simulink model "TST_AccPed_DrvDemStpLim"  (R2016b)
settings: Solver=FixedStepDiscrete  StartTime=0.0  StopTime=simTime  FixedStep=sampleTime  RelTol=1e-3
values from neighbouring files (symbols this model uses):
  testCase = 1    [initTST_AccPed_DrvDemStpLim_001.m]    (also in initTST_AccPed_DrvDemStpLim_002.m = 2; initTST_AccPed_DrvDemStpLim_003.m = 3)
libraries: simulink x13, UnitTest_Lib x9
settings Model: Creator=zhengjinyan  LastModifiedBy=zhengjinyan
settings DebuggingCC: SignalRangeChecking=error

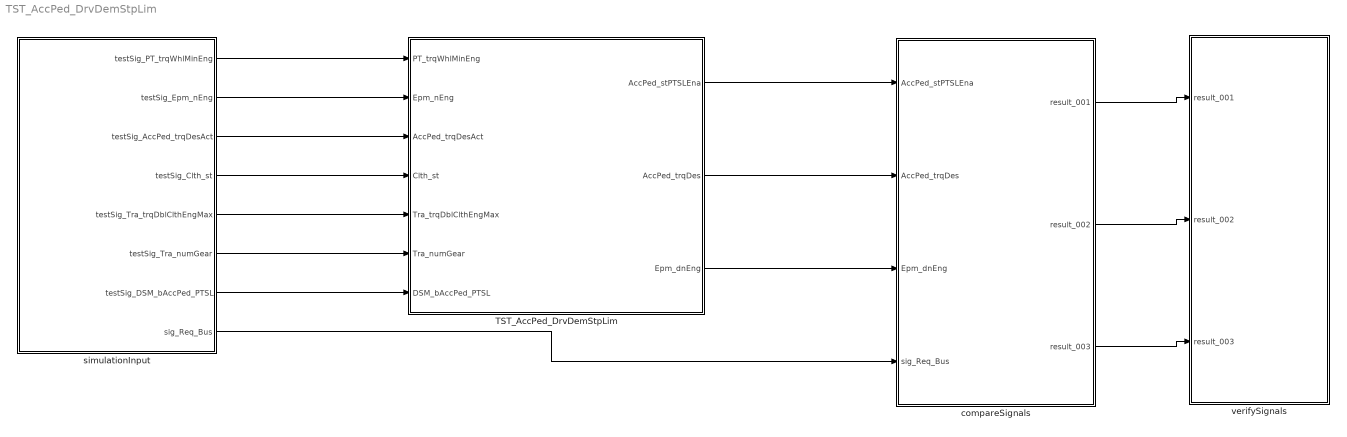
== system TST_AccPed_DrvDemStpLim ==
  TST_AccPed_DrvDemStpLim : Subsystem
  compareSignals : Subsystem
  simulationInput : Subsystem
  verifySignals : Subsystem
  wires:
  simulationInput/1(testSig_PT_trqWhlMinEng) -> TST_AccPed_DrvDemStpLim/1(PT_trqWhlMinEng)
  simulationInput/2(testSig_Epm_nEng) -> TST_AccPed_DrvDemStpLim/2(Epm_nEng)
  simulationInput/3(testSig_AccPed_trqDesAct) -> TST_AccPed_DrvDemStpLim/3(AccPed_trqDesAct)
  simulationInput/4(testSig_Clth_st) -> TST_AccPed_DrvDemStpLim/4(Clth_st)
  simulationInput/5(testSig_Tra_trqDblClthEngMax) -> TST_AccPed_DrvDemStpLim/5(Tra_trqDblClthEngMax)
  simulationInput/6(testSig_Tra_numGear) -> TST_AccPed_DrvDemStpLim/6(Tra_numGear)
  simulationInput/7(testSig_DSM_bAccPed_PTSL) -> TST_AccPed_DrvDemStpLim/7(DSM_bAccPed_PTSL)
  TST_AccPed_DrvDemStpLim/1(AccPed_stPTSLEna) -> compareSignals/1(AccPed_stPTSLEna)
  TST_AccPed_DrvDemStpLim/2(AccPed_trqDes) -> compareSignals/2(AccPed_trqDes)
  TST_AccPed_DrvDemStpLim/3(Epm_dnEng) -> compareSignals/3(Epm_dnEng)
  simulationInput/8(sig_Req_Bus) -> compareSignals/4(sig_Req_Bus)
  compareSignals/1(result_001) -> verifySignals/1(result_001)
  compareSignals/2(result_002) -> verifySignals/2(result_002)
  compareSignals/3(result_003) -> verifySignals/3(result_003)

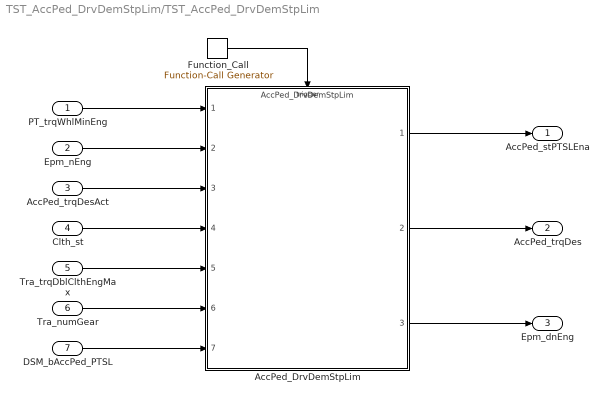
== system TST_AccPed_DrvDemStpLim/TST_AccPed_DrvDemStpLim ==
  PT_trqWhlMinEng : Inport
  Epm_nEng : Inport  Port=2
  AccPed_trqDesAct : Inport  Port=3
  Clth_st : Inport  Port=4
  Tra_trqDblClthEngMax : Inport  Port=5
  Tra_numGear : Inport  Port=6
  DSM_bAccPed_PTSL : Inport  Port=7
  AccPed_DrvDemStpLim : ModelReference  ModelNameDialog=AccPed_DrvDemStpLim  SimulationMode=Normal  ModelReferenceVersion=1.9  TriggerPortName=function  TriggerPortTriggerType=function-call  TriggerPortStatesWhenEnabling=held
  Function_Call : simulink/Ports & Subsystems/Function-Call Generator  sample_time=sampleTime  numberOfIterations=1
  AccPed_stPTSLEna : Outport
  AccPed_trqDes : Outport  Port=2
  Epm_dnEng : Outport  Port=3
  wires:
  Function_Call/1 -> AccPed_DrvDemStpLim/Trigger
  PT_trqWhlMinEng/1 -> AccPed_DrvDemStpLim/1
  Epm_nEng/1 -> AccPed_DrvDemStpLim/2
  AccPed_trqDesAct/1 -> AccPed_DrvDemStpLim/3
  Clth_st/1 -> AccPed_DrvDemStpLim/4
  Tra_trqDblClthEngMax/1 -> AccPed_DrvDemStpLim/5
  Tra_numGear/1 -> AccPed_DrvDemStpLim/6
  DSM_bAccPed_PTSL/1 -> AccPed_DrvDemStpLim/7
  AccPed_DrvDemStpLim/1 -> AccPed_stPTSLEna/1
  AccPed_DrvDemStpLim/2 -> AccPed_trqDes/1
  AccPed_DrvDemStpLim/3 -> Epm_dnEng/1

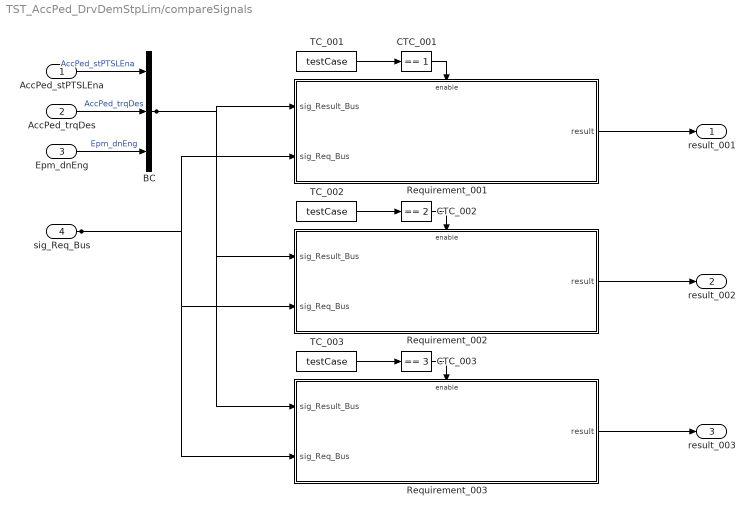
== system TST_AccPed_DrvDemStpLim/compareSignals ==
  AccPed_stPTSLEna : Inport
  AccPed_trqDes : Inport  Port=2
  Epm_dnEng : Inport  Port=3
  sig_Req_Bus : Inport  Port=4
  BC : BusCreator  Inputs=3
  CTC_001 : simulink/Logic and Bit Operations/Compare To Constant  relop===  const=1  OutDataTypeStr=boolean
  CTC_002 : simulink/Logic and Bit Operations/Compare To Constant  relop===  const=2  OutDataTypeStr=boolean
  CTC_003 : simulink/Logic and Bit Operations/Compare To Constant  relop===  const=3  OutDataTypeStr=boolean
  Requirement_001 : Subsystem
  Requirement_002 : Subsystem
  Requirement_003 : Subsystem
  TC_001 : Constant  Value=testCase
  TC_002 : Constant  Value=testCase
  TC_003 : Constant  Value=testCase
  result_001 : Outport
  result_002 : Outport  Port=2
  result_003 : Outport  Port=3
  wires:
  AccPed_stPTSLEna/1 -> BC/1  "AccPed_stPTSLEna"
  AccPed_trqDes/1 -> BC/2  "AccPed_trqDes"
  Epm_dnEng/1 -> BC/3  "Epm_dnEng"
  TC_001/1 -> CTC_001/1
  CTC_001/1 -> Requirement_001/Enable
  sig_Req_Bus/1 -> Requirement_001/2(sig_Req_Bus), Requirement_002/2(sig_Req_Bus), Requirement_003/2(sig_Req_Bus)
  BC/1 -> Requirement_001/1(sig_Result_Bus), Requirement_002/1(sig_Result_Bus), Requirement_003/1(sig_Result_Bus)
  Requirement_001/1(result) -> result_001/1
  TC_002/1 -> CTC_002/1
  CTC_002/1 -> Requirement_002/Enable
  Requirement_002/1(result) -> result_002/1
  TC_003/1 -> CTC_003/1
  CTC_003/1 -> Requirement_003/Enable
  Requirement_003/1(result) -> result_003/1

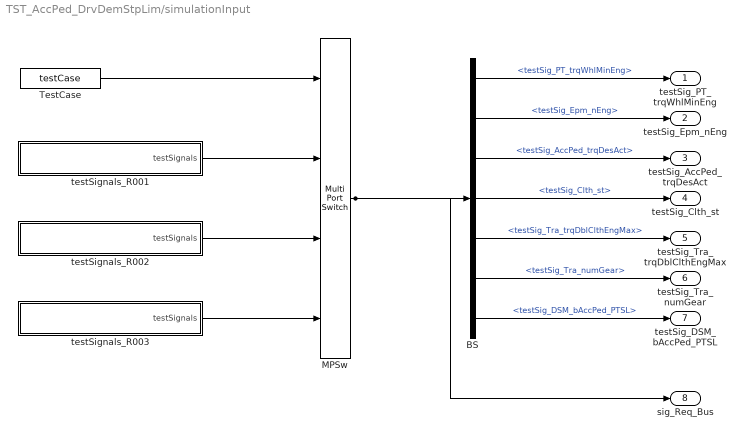
== system TST_AccPed_DrvDemStpLim/simulationInput ==
  BS : BusSelector  OutputSignals=testSig_PT_trqWhlMinEng,testSig_Epm_nEng,testSig_AccPed_trqDesAct,testSig_Clth_st,testSig_Tra_trqDblClthEngMax,testSig_Tra_numGear,testSig_DSM_bAccPed_PTSL
  MPSw : MultiPortSwitch  SaturateOnIntegerOverflow=on  InputSameDT=on
  TestCase : Constant  Value=testCase
  testSignals_R001 : Subsystem
  testSignals_R002 : Subsystem
  testSignals_R003 : Subsystem
  testSig_PT_trqWhlMinEng : Outport
  testSig_Epm_nEng : Outport  Port=2
  testSig_AccPed_trqDesAct : Outport  Port=3
  testSig_Clth_st : Outport  Port=4
  testSig_Tra_trqDblClthEngMax : Outport  Port=5
  testSig_Tra_numGear : Outport  Port=6
  testSig_DSM_bAccPed_PTSL : Outport  Port=7
  sig_Req_Bus : Outport  Port=8
  wires:
  BS/1 -> testSig_PT_trqWhlMinEng/1  "<testSig_PT_trqWhlMinEng>"
  BS/2 -> testSig_Epm_nEng/1  "<testSig_Epm_nEng>"
  BS/3 -> testSig_AccPed_trqDesAct/1  "<testSig_AccPed_trqDesAct>"
  BS/4 -> testSig_Clth_st/1  "<testSig_Clth_st>"
  BS/5 -> testSig_Tra_trqDblClthEngMax/1  "<testSig_Tra_trqDblClthEngMax>"
  BS/6 -> testSig_Tra_numGear/1  "<testSig_Tra_numGear>"
  BS/7 -> testSig_DSM_bAccPed_PTSL/1  "<testSig_DSM_bAccPed_PTSL>"
  MPSw/1 -> BS/1, sig_Req_Bus/1
  TestCase/1 -> MPSw/1
  testSignals_R001/1(testSignals) -> MPSw/2
  testSignals_R002/1(testSignals) -> MPSw/3
  testSignals_R003/1(testSignals) -> MPSw/4

== system TST_AccPed_DrvDemStpLim/verifySignals ==
  result_001 : Inport
  result_002 : Inport  Port=2
  result_003 : Inport  Port=3
  Assertion_001 : Assertion  Enabled=off
  Assertion_002 : Assertion  Enabled=off
  Assertion_003 : Assertion  Enabled=off
  wires:
  result_001/1 -> Assertion_001/1
  result_002/1 -> Assertion_002/1
  result_003/1 -> Assertion_003/1

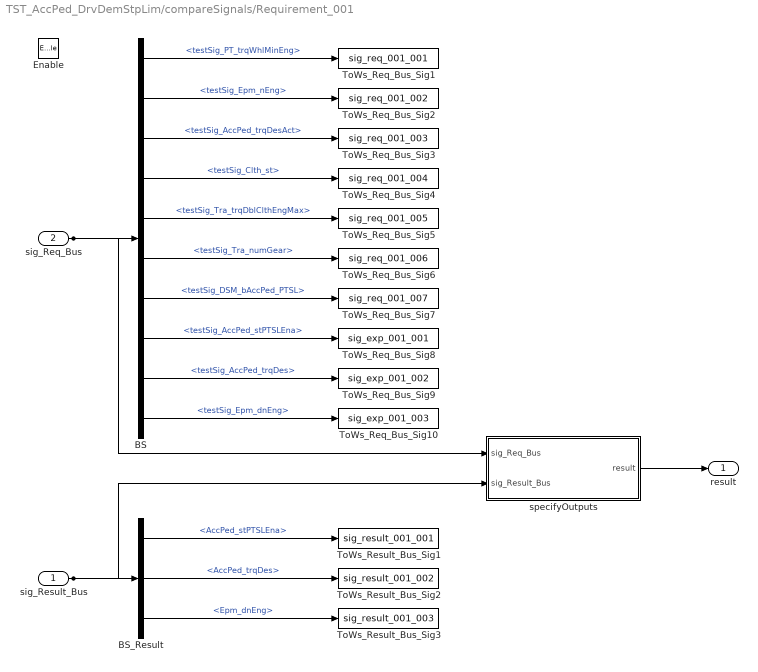
== system TST_AccPed_DrvDemStpLim/compareSignals/Requirement_001 ==
  sig_Result_Bus : Inport
  sig_Req_Bus : Inport  Port=2
  Enable : EnablePort
  BS : BusSelector  OutputSignals=testSig_PT_trqWhlMinEng,testSig_Epm_nEng,testSig_AccPed_trqDesAct,testSig_Clth_st,testSig_Tra_trqDblClthEngMax,testSig_Tra_numGear,testSig_DSM_bAccPed_PTSL,testSig_AccPed_stPTSLEna,testSig_AccPed_trqDes,testSig_Epm_dnEng
  BS_Result : BusSelector  OutputSignals=AccPed_stPTSLEna,AccPed_trqDes,Epm_dnEng
  ToWs_Req_Bus_Sig1 : ToWorkspace  VariableName=sig_req_001_001  SaveFormat=Structure With Time
  ToWs_Req_Bus_Sig10 : ToWorkspace  VariableName=sig_exp_001_003  SaveFormat=Structure With Time
  ToWs_Req_Bus_Sig2 : ToWorkspace  VariableName=sig_req_001_002  SaveFormat=Structure With Time
  ToWs_Req_Bus_Sig3 : ToWorkspace  VariableName=sig_req_001_003  SaveFormat=Structure With Time
  ToWs_Req_Bus_Sig4 : ToWorkspace  VariableName=sig_req_001_004  SaveFormat=Structure With Time
  ToWs_Req_Bus_Sig5 : ToWorkspace  VariableName=sig_req_001_005  SaveFormat=Structure With Time
  ToWs_Req_Bus_Sig6 : ToWorkspace  VariableName=sig_req_001_006  SaveFormat=Structure With Time
  ToWs_Req_Bus_Sig7 : ToWorkspace  VariableName=sig_req_001_007  SaveFormat=Structure With Time
  ToWs_Req_Bus_Sig8 : ToWorkspace  VariableName=sig_exp_001_001  SaveFormat=Structure With Time
  ToWs_Req_Bus_Sig9 : ToWorkspace  VariableName=sig_exp_001_002  SaveFormat=Structure With Time
  ToWs_Result_Bus_Sig1 : ToWorkspace  VariableName=sig_result_001_001  SaveFormat=Structure With Time
  ToWs_Result_Bus_Sig2 : ToWorkspace  VariableName=sig_result_001_002  SaveFormat=Structure With Time
  ToWs_Result_Bus_Sig3 : ToWorkspace  VariableName=sig_result_001_003  SaveFormat=Structure With Time
  specifyOutputs : Subsystem
  result : Outport
  wires:
  sig_Req_Bus/1 -> BS/1, specifyOutputs/1(sig_Req_Bus)
  BS/1 -> ToWs_Req_Bus_Sig1/1  "<testSig_PT_trqWhlMinEng>"
  BS/2 -> ToWs_Req_Bus_Sig2/1  "<testSig_Epm_nEng>"
  BS/3 -> ToWs_Req_Bus_Sig3/1  "<testSig_AccPed_trqDesAct>"
  BS/4 -> ToWs_Req_Bus_Sig4/1  "<testSig_Clth_st>"
  BS/5 -> ToWs_Req_Bus_Sig5/1  "<testSig_Tra_trqDblClthEngMax>"
  BS/6 -> ToWs_Req_Bus_Sig6/1  "<testSig_Tra_numGear>"
  BS/7 -> ToWs_Req_Bus_Sig7/1  "<testSig_DSM_bAccPed_PTSL>"
  BS/8 -> ToWs_Req_Bus_Sig8/1  "<testSig_AccPed_stPTSLEna>"
  BS/9 -> ToWs_Req_Bus_Sig9/1  "<testSig_AccPed_trqDes>"
  BS/10 -> ToWs_Req_Bus_Sig10/1  "<testSig_Epm_dnEng>"
  sig_Result_Bus/1 -> BS_Result/1, specifyOutputs/2(sig_Result_Bus)
  BS_Result/1 -> ToWs_Result_Bus_Sig1/1  "<AccPed_stPTSLEna>"
  BS_Result/2 -> ToWs_Result_Bus_Sig2/1  "<AccPed_trqDes>"
  BS_Result/3 -> ToWs_Result_Bus_Sig3/1  "<Epm_dnEng>"
  specifyOutputs/1(result) -> result/1

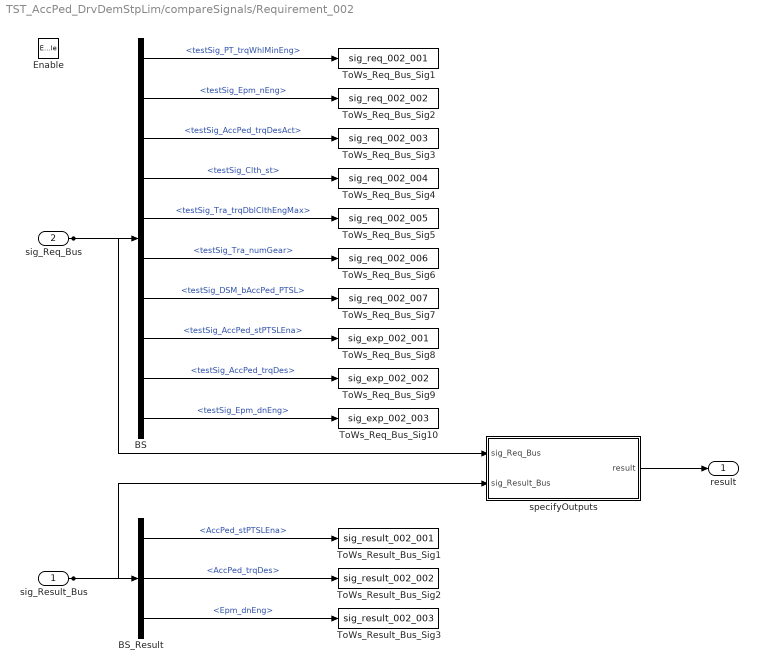
== system TST_AccPed_DrvDemStpLim/compareSignals/Requirement_002 ==
  sig_Result_Bus : Inport
  sig_Req_Bus : Inport  Port=2
  Enable : EnablePort
  BS : BusSelector  OutputSignals=testSig_PT_trqWhlMinEng,testSig_Epm_nEng,testSig_AccPed_trqDesAct,testSig_Clth_st,testSig_Tra_trqDblClthEngMax,testSig_Tra_numGear,testSig_DSM_bAccPed_PTSL,testSig_AccPed_stPTSLEna,testSig_AccPed_trqDes,testSig_Epm_dnEng
  BS_Result : BusSelector  OutputSignals=AccPed_stPTSLEna,AccPed_trqDes,Epm_dnEng
  ToWs_Req_Bus_Sig1 : ToWorkspace  VariableName=sig_req_002_001  SaveFormat=Structure With Time
  ToWs_Req_Bus_Sig10 : ToWorkspace  VariableName=sig_exp_002_003  SaveFormat=Structure With Time
  ToWs_Req_Bus_Sig2 : ToWorkspace  VariableName=sig_req_002_002  SaveFormat=Structure With Time
  ToWs_Req_Bus_Sig3 : ToWorkspace  VariableName=sig_req_002_003  SaveFormat=Structure With Time
  ToWs_Req_Bus_Sig4 : ToWorkspace  VariableName=sig_req_002_004  SaveFormat=Structure With Time
  ToWs_Req_Bus_Sig5 : ToWorkspace  VariableName=sig_req_002_005  SaveFormat=Structure With Time
  ToWs_Req_Bus_Sig6 : ToWorkspace  VariableName=sig_req_002_006  SaveFormat=Structure With Time
  ToWs_Req_Bus_Sig7 : ToWorkspace  VariableName=sig_req_002_007  SaveFormat=Structure With Time
  ToWs_Req_Bus_Sig8 : ToWorkspace  VariableName=sig_exp_002_001  SaveFormat=Structure With Time
  ToWs_Req_Bus_Sig9 : ToWorkspace  VariableName=sig_exp_002_002  SaveFormat=Structure With Time
  ToWs_Result_Bus_Sig1 : ToWorkspace  VariableName=sig_result_002_001  SaveFormat=Structure With Time
  ToWs_Result_Bus_Sig2 : ToWorkspace  VariableName=sig_result_002_002  SaveFormat=Structure With Time
  ToWs_Result_Bus_Sig3 : ToWorkspace  VariableName=sig_result_002_003  SaveFormat=Structure With Time
  specifyOutputs : Subsystem
  result : Outport
  wires:
  sig_Req_Bus/1 -> BS/1, specifyOutputs/1(sig_Req_Bus)
  BS/1 -> ToWs_Req_Bus_Sig1/1  "<testSig_PT_trqWhlMinEng>"
  BS/2 -> ToWs_Req_Bus_Sig2/1  "<testSig_Epm_nEng>"
  BS/3 -> ToWs_Req_Bus_Sig3/1  "<testSig_AccPed_trqDesAct>"
  BS/4 -> ToWs_Req_Bus_Sig4/1  "<testSig_Clth_st>"
  BS/5 -> ToWs_Req_Bus_Sig5/1  "<testSig_Tra_trqDblClthEngMax>"
  BS/6 -> ToWs_Req_Bus_Sig6/1  "<testSig_Tra_numGear>"
  BS/7 -> ToWs_Req_Bus_Sig7/1  "<testSig_DSM_bAccPed_PTSL>"
  BS/8 -> ToWs_Req_Bus_Sig8/1  "<testSig_AccPed_stPTSLEna>"
  BS/9 -> ToWs_Req_Bus_Sig9/1  "<testSig_AccPed_trqDes>"
  BS/10 -> ToWs_Req_Bus_Sig10/1  "<testSig_Epm_dnEng>"
  sig_Result_Bus/1 -> BS_Result/1, specifyOutputs/2(sig_Result_Bus)
  BS_Result/1 -> ToWs_Result_Bus_Sig1/1  "<AccPed_stPTSLEna>"
  BS_Result/2 -> ToWs_Result_Bus_Sig2/1  "<AccPed_trqDes>"
  BS_Result/3 -> ToWs_Result_Bus_Sig3/1  "<Epm_dnEng>"
  specifyOutputs/1(result) -> result/1

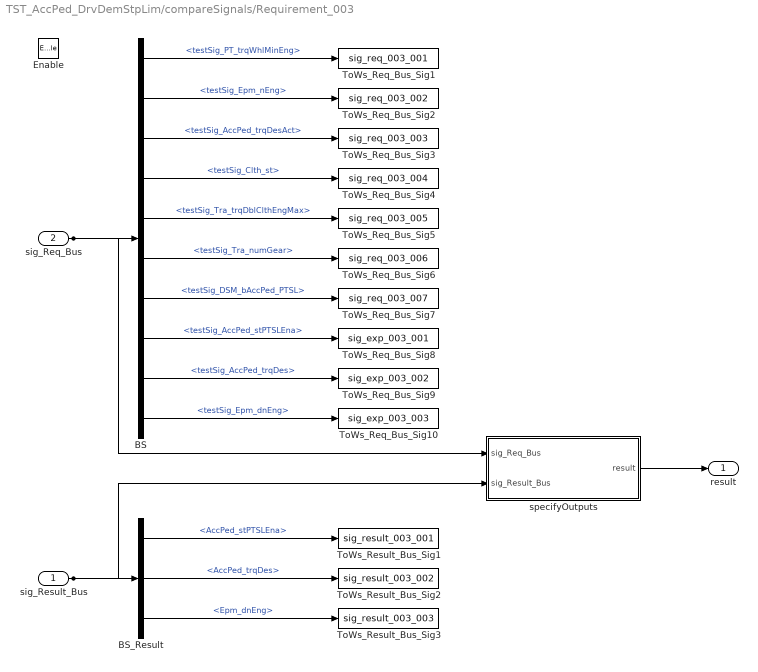
== system TST_AccPed_DrvDemStpLim/compareSignals/Requirement_003 ==
  sig_Result_Bus : Inport
  sig_Req_Bus : Inport  Port=2
  Enable : EnablePort
  BS : BusSelector  OutputSignals=testSig_PT_trqWhlMinEng,testSig_Epm_nEng,testSig_AccPed_trqDesAct,testSig_Clth_st,testSig_Tra_trqDblClthEngMax,testSig_Tra_numGear,testSig_DSM_bAccPed_PTSL,testSig_AccPed_stPTSLEna,testSig_AccPed_trqDes,testSig_Epm_dnEng
  BS_Result : BusSelector  OutputSignals=AccPed_stPTSLEna,AccPed_trqDes,Epm_dnEng
  ToWs_Req_Bus_Sig1 : ToWorkspace  VariableName=sig_req_003_001  SaveFormat=Structure With Time
  ToWs_Req_Bus_Sig10 : ToWorkspace  VariableName=sig_exp_003_003  SaveFormat=Structure With Time
  ToWs_Req_Bus_Sig2 : ToWorkspace  VariableName=sig_req_003_002  SaveFormat=Structure With Time
  ToWs_Req_Bus_Sig3 : ToWorkspace  VariableName=sig_req_003_003  SaveFormat=Structure With Time
  ToWs_Req_Bus_Sig4 : ToWorkspace  VariableName=sig_req_003_004  SaveFormat=Structure With Time
  ToWs_Req_Bus_Sig5 : ToWorkspace  VariableName=sig_req_003_005  SaveFormat=Structure With Time
  ToWs_Req_Bus_Sig6 : ToWorkspace  VariableName=sig_req_003_006  SaveFormat=Structure With Time
  ToWs_Req_Bus_Sig7 : ToWorkspace  VariableName=sig_req_003_007  SaveFormat=Structure With Time
  ToWs_Req_Bus_Sig8 : ToWorkspace  VariableName=sig_exp_003_001  SaveFormat=Structure With Time
  ToWs_Req_Bus_Sig9 : ToWorkspace  VariableName=sig_exp_003_002  SaveFormat=Structure With Time
  ToWs_Result_Bus_Sig1 : ToWorkspace  VariableName=sig_result_003_001  SaveFormat=Structure With Time
  ToWs_Result_Bus_Sig2 : ToWorkspace  VariableName=sig_result_003_002  SaveFormat=Structure With Time
  ToWs_Result_Bus_Sig3 : ToWorkspace  VariableName=sig_result_003_003  SaveFormat=Structure With Time
  specifyOutputs : Subsystem
  result : Outport
  wires:
  sig_Req_Bus/1 -> BS/1, specifyOutputs/1(sig_Req_Bus)
  BS/1 -> ToWs_Req_Bus_Sig1/1  "<testSig_PT_trqWhlMinEng>"
  BS/2 -> ToWs_Req_Bus_Sig2/1  "<testSig_Epm_nEng>"
  BS/3 -> ToWs_Req_Bus_Sig3/1  "<testSig_AccPed_trqDesAct>"
  BS/4 -> ToWs_Req_Bus_Sig4/1  "<testSig_Clth_st>"
  BS/5 -> ToWs_Req_Bus_Sig5/1  "<testSig_Tra_trqDblClthEngMax>"
  BS/6 -> ToWs_Req_Bus_Sig6/1  "<testSig_Tra_numGear>"
  BS/7 -> ToWs_Req_Bus_Sig7/1  "<testSig_DSM_bAccPed_PTSL>"
  BS/8 -> ToWs_Req_Bus_Sig8/1  "<testSig_AccPed_stPTSLEna>"
  BS/9 -> ToWs_Req_Bus_Sig9/1  "<testSig_AccPed_trqDes>"
  BS/10 -> ToWs_Req_Bus_Sig10/1  "<testSig_Epm_dnEng>"
  sig_Result_Bus/1 -> BS_Result/1, specifyOutputs/2(sig_Result_Bus)
  BS_Result/1 -> ToWs_Result_Bus_Sig1/1  "<AccPed_stPTSLEna>"
  BS_Result/2 -> ToWs_Result_Bus_Sig2/1  "<AccPed_trqDes>"
  BS_Result/3 -> ToWs_Result_Bus_Sig3/1  "<Epm_dnEng>"
  specifyOutputs/1(result) -> result/1

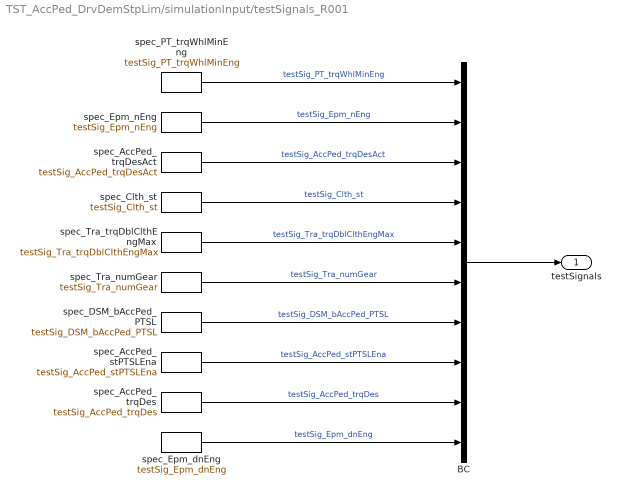
== system TST_AccPed_DrvDemStpLim/simulationInput/testSignals_R001 ==
  BC : BusCreator  Inputs=10
  spec_AccPed_stPTSLEna : FromWorkspace  VariableName=testSig_AccPed_stPTSLEna  Interpolate=off  OutputAfterFinalValue=Holding final value
  spec_AccPed_trqDes : FromWorkspace  VariableName=testSig_AccPed_trqDes  Interpolate=off  OutputAfterFinalValue=Holding final value
  spec_AccPed_trqDesAct : FromWorkspace  VariableName=testSig_AccPed_trqDesAct  Interpolate=off  OutputAfterFinalValue=Holding final value
  spec_Clth_st : FromWorkspace  VariableName=testSig_Clth_st  Interpolate=off  OutputAfterFinalValue=Holding final value
  spec_DSM_bAccPed_PTSL : FromWorkspace  VariableName=testSig_DSM_bAccPed_PTSL  Interpolate=off  OutputAfterFinalValue=Holding final value
  spec_Epm_dnEng : FromWorkspace  VariableName=testSig_Epm_dnEng  Interpolate=off  OutputAfterFinalValue=Holding final value
  spec_Epm_nEng : FromWorkspace  VariableName=testSig_Epm_nEng  Interpolate=off  OutputAfterFinalValue=Holding final value
  spec_PT_trqWhlMinEng : FromWorkspace  VariableName=testSig_PT_trqWhlMinEng  Interpolate=off  OutputAfterFinalValue=Holding final value
  spec_Tra_numGear : FromWorkspace  VariableName=testSig_Tra_numGear  Interpolate=off  OutputAfterFinalValue=Holding final value
  spec_Tra_trqDblClthEngMax : FromWorkspace  VariableName=testSig_Tra_trqDblClthEngMax  Interpolate=off  OutputAfterFinalValue=Holding final value
  testSignals : Outport
  wires:
  BC/1 -> testSignals/1
  spec_PT_trqWhlMinEng/1 -> BC/1  "testSig_PT_trqWhlMinEng"
  spec_Epm_nEng/1 -> BC/2  "testSig_Epm_nEng"
  spec_AccPed_trqDesAct/1 -> BC/3  "testSig_AccPed_trqDesAct"
  spec_Clth_st/1 -> BC/4  "testSig_Clth_st"
  spec_Tra_trqDblClthEngMax/1 -> BC/5  "testSig_Tra_trqDblClthEngMax"
  spec_Tra_numGear/1 -> BC/6  "testSig_Tra_numGear"
  spec_DSM_bAccPed_PTSL/1 -> BC/7  "testSig_DSM_bAccPed_PTSL"
  spec_AccPed_stPTSLEna/1 -> BC/8  "testSig_AccPed_stPTSLEna"
  spec_AccPed_trqDes/1 -> BC/9  "testSig_AccPed_trqDes"
  spec_Epm_dnEng/1 -> BC/10  "testSig_Epm_dnEng"

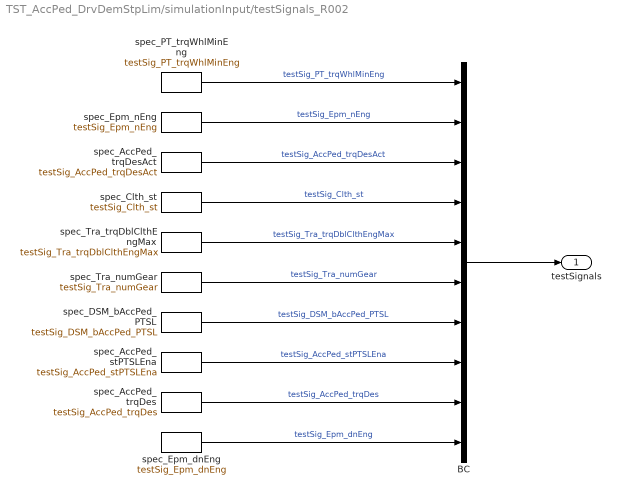
== system TST_AccPed_DrvDemStpLim/simulationInput/testSignals_R002 ==
  BC : BusCreator  Inputs=10
  spec_AccPed_stPTSLEna : FromWorkspace  VariableName=testSig_AccPed_stPTSLEna  Interpolate=off  OutputAfterFinalValue=Holding final value
  spec_AccPed_trqDes : FromWorkspace  VariableName=testSig_AccPed_trqDes  Interpolate=off  OutputAfterFinalValue=Holding final value
  spec_AccPed_trqDesAct : FromWorkspace  VariableName=testSig_AccPed_trqDesAct  Interpolate=off  OutputAfterFinalValue=Holding final value
  spec_Clth_st : FromWorkspace  VariableName=testSig_Clth_st  Interpolate=off  OutputAfterFinalValue=Holding final value
  spec_DSM_bAccPed_PTSL : FromWorkspace  VariableName=testSig_DSM_bAccPed_PTSL  Interpolate=off  OutputAfterFinalValue=Holding final value
  spec_Epm_dnEng : FromWorkspace  VariableName=testSig_Epm_dnEng  Interpolate=off  OutputAfterFinalValue=Holding final value
  spec_Epm_nEng : FromWorkspace  VariableName=testSig_Epm_nEng  Interpolate=off  OutputAfterFinalValue=Holding final value
  spec_PT_trqWhlMinEng : FromWorkspace  VariableName=testSig_PT_trqWhlMinEng  Interpolate=off  OutputAfterFinalValue=Holding final value
  spec_Tra_numGear : FromWorkspace  VariableName=testSig_Tra_numGear  Interpolate=off  OutputAfterFinalValue=Holding final value
  spec_Tra_trqDblClthEngMax : FromWorkspace  VariableName=testSig_Tra_trqDblClthEngMax  Interpolate=off  OutputAfterFinalValue=Holding final value
  testSignals : Outport
  wires:
  BC/1 -> testSignals/1
  spec_PT_trqWhlMinEng/1 -> BC/1  "testSig_PT_trqWhlMinEng"
  spec_Epm_nEng/1 -> BC/2  "testSig_Epm_nEng"
  spec_AccPed_trqDesAct/1 -> BC/3  "testSig_AccPed_trqDesAct"
  spec_Clth_st/1 -> BC/4  "testSig_Clth_st"
  spec_Tra_trqDblClthEngMax/1 -> BC/5  "testSig_Tra_trqDblClthEngMax"
  spec_Tra_numGear/1 -> BC/6  "testSig_Tra_numGear"
  spec_DSM_bAccPed_PTSL/1 -> BC/7  "testSig_DSM_bAccPed_PTSL"
  spec_AccPed_stPTSLEna/1 -> BC/8  "testSig_AccPed_stPTSLEna"
  spec_AccPed_trqDes/1 -> BC/9  "testSig_AccPed_trqDes"
  spec_Epm_dnEng/1 -> BC/10  "testSig_Epm_dnEng"

== system TST_AccPed_DrvDemStpLim/simulationInput/testSignals_R003 ==
  BC : BusCreator  Inputs=10
  spec_AccPed_stPTSLEna : FromWorkspace  VariableName=testSig_AccPed_stPTSLEna  Interpolate=off  OutputAfterFinalValue=Holding final value
  spec_AccPed_trqDes : FromWorkspace  VariableName=testSig_AccPed_trqDes  Interpolate=off  OutputAfterFinalValue=Holding final value
  spec_AccPed_trqDesAct : FromWorkspace  VariableName=testSig_AccPed_trqDesAct  Interpolate=off  OutputAfterFinalValue=Holding final value
  spec_Clth_st : FromWorkspace  VariableName=testSig_Clth_st  Interpolate=off  OutputAfterFinalValue=Holding final value
  spec_DSM_bAccPed_PTSL : FromWorkspace  VariableName=testSig_DSM_bAccPed_PTSL  Interpolate=off  OutputAfterFinalValue=Holding final value
  spec_Epm_dnEng : FromWorkspace  VariableName=testSig_Epm_dnEng  Interpolate=off  OutputAfterFinalValue=Holding final value
  spec_Epm_nEng : FromWorkspace  VariableName=testSig_Epm_nEng  Interpolate=off  OutputAfterFinalValue=Holding final value
  spec_PT_trqWhlMinEng : FromWorkspace  VariableName=testSig_PT_trqWhlMinEng  Interpolate=off  OutputAfterFinalValue=Holding final value
  spec_Tra_numGear : FromWorkspace  VariableName=testSig_Tra_numGear  Interpolate=off  OutputAfterFinalValue=Holding final value
  spec_Tra_trqDblClthEngMax : FromWorkspace  VariableName=testSig_Tra_trqDblClthEngMax  Interpolate=off  OutputAfterFinalValue=Holding final value
  testSignals : Outport
  wires:
  BC/1 -> testSignals/1
  spec_PT_trqWhlMinEng/1 -> BC/1  "testSig_PT_trqWhlMinEng"
  spec_Epm_nEng/1 -> BC/2  "testSig_Epm_nEng"
  spec_AccPed_trqDesAct/1 -> BC/3  "testSig_AccPed_trqDesAct"
  spec_Clth_st/1 -> BC/4  "testSig_Clth_st"
  spec_Tra_trqDblClthEngMax/1 -> BC/5  "testSig_Tra_trqDblClthEngMax"
  spec_Tra_numGear/1 -> BC/6  "testSig_Tra_numGear"
  spec_DSM_bAccPed_PTSL/1 -> BC/7  "testSig_DSM_bAccPed_PTSL"
  spec_AccPed_stPTSLEna/1 -> BC/8  "testSig_AccPed_stPTSLEna"
  spec_AccPed_trqDes/1 -> BC/9  "testSig_AccPed_trqDes"
  spec_Epm_dnEng/1 -> BC/10  "testSig_Epm_dnEng"

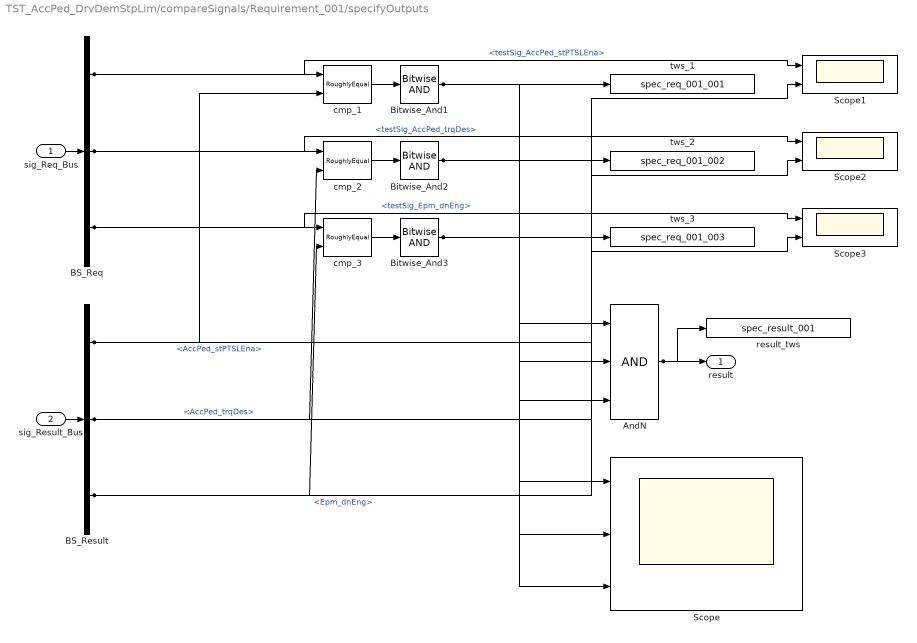
== system TST_AccPed_DrvDemStpLim/compareSignals/Requirement_001/specifyOutputs ==
  sig_Req_Bus : Inport
  sig_Result_Bus : Inport  Port=2
  AndN : Logic  Inputs=3
  BS_Req : BusSelector  OutputSignals=testSig_AccPed_stPTSLEna,testSig_AccPed_trqDes,testSig_Epm_dnEng
  BS_Result : BusSelector  OutputSignals=AccPed_stPTSLEna,AccPed_trqDes,Epm_dnEng
  Bitwise_And1 : simulink/Logic and Bit Operations/Bitwise Operator  logicop=AND  UseBitMask=off  BitMask=bin2dec('11011001')  BitMaskRealWorld=Stored Integer
  Bitwise_And2 : simulink/Logic and Bit Operations/Bitwise Operator  logicop=AND  UseBitMask=off  BitMask=bin2dec('11011001')  BitMaskRealWorld=Stored Integer
  Bitwise_And3 : simulink/Logic and Bit Operations/Bitwise Operator  logicop=AND  UseBitMask=off  BitMask=bin2dec('11011001')  BitMaskRealWorld=Stored Integer
  Scope : Scope  NumInputPorts=3
  Scope1 : Scope  NumInputPorts=2
  Scope2 : Scope  NumInputPorts=2
  Scope3 : Scope  NumInputPorts=2
  cmp_1 : UnitTest_Lib/RoughlyEqual  slope=0.1
  cmp_2 : UnitTest_Lib/RoughlyEqual  slope=0.1
  cmp_3 : UnitTest_Lib/RoughlyEqual  slope=0.1
  result_tws : ToWorkspace  VariableName=spec_result_001
  tws_1 : ToWorkspace  VariableName=spec_req_001_001
  tws_2 : ToWorkspace  VariableName=spec_req_001_002
  tws_3 : ToWorkspace  VariableName=spec_req_001_003
  result : Outport
  wires:
  sig_Req_Bus/1 -> BS_Req/1
  sig_Result_Bus/1 -> BS_Result/1
  AndN/1 -> result/1, result_tws/1
  BS_Req/1 -> cmp_1/1, Scope1/1  "<testSig_AccPed_stPTSLEna>"
  BS_Result/1 -> cmp_1/2, Scope1/2  "<AccPed_stPTSLEna>"
  cmp_1/1 -> Bitwise_And1/1
  Bitwise_And1/1 -> tws_1/1, AndN/1, Scope/1
  BS_Req/2 -> cmp_2/1, Scope2/1  "<testSig_AccPed_trqDes>"
  BS_Result/2 -> cmp_2/2, Scope2/2  "<AccPed_trqDes>"
  cmp_2/1 -> Bitwise_And2/1
  Bitwise_And2/1 -> tws_2/1, AndN/2, Scope/2
  BS_Req/3 -> cmp_3/1, Scope3/1  "<testSig_Epm_dnEng>"
  BS_Result/3 -> cmp_3/2, Scope3/2  "<Epm_dnEng>"
  cmp_3/1 -> Bitwise_And3/1
  Bitwise_And3/1 -> tws_3/1, AndN/3, Scope/3

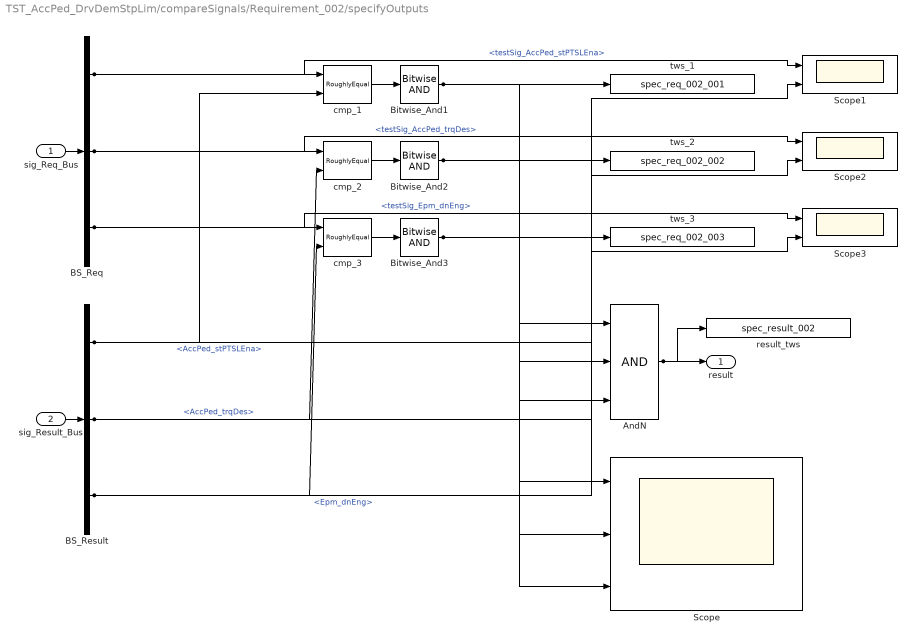
== system TST_AccPed_DrvDemStpLim/compareSignals/Requirement_002/specifyOutputs ==
  sig_Req_Bus : Inport
  sig_Result_Bus : Inport  Port=2
  AndN : Logic  Inputs=3
  BS_Req : BusSelector  OutputSignals=testSig_AccPed_stPTSLEna,testSig_AccPed_trqDes,testSig_Epm_dnEng
  BS_Result : BusSelector  OutputSignals=AccPed_stPTSLEna,AccPed_trqDes,Epm_dnEng
  Bitwise_And1 : simulink/Logic and Bit Operations/Bitwise Operator  logicop=AND  UseBitMask=off  BitMask=bin2dec('11011001')  BitMaskRealWorld=Stored Integer
  Bitwise_And2 : simulink/Logic and Bit Operations/Bitwise Operator  logicop=AND  UseBitMask=off  BitMask=bin2dec('11011001')  BitMaskRealWorld=Stored Integer
  Bitwise_And3 : simulink/Logic and Bit Operations/Bitwise Operator  logicop=AND  UseBitMask=off  BitMask=bin2dec('11011001')  BitMaskRealWorld=Stored Integer
  Scope : Scope  NumInputPorts=3
  Scope1 : Scope  NumInputPorts=2
  Scope2 : Scope  NumInputPorts=2
  Scope3 : Scope  NumInputPorts=2
  cmp_1 : UnitTest_Lib/RoughlyEqual  slope=0.1
  cmp_2 : UnitTest_Lib/RoughlyEqual  slope=0.1
  cmp_3 : UnitTest_Lib/RoughlyEqual  slope=0.1
  result_tws : ToWorkspace  VariableName=spec_result_002
  tws_1 : ToWorkspace  VariableName=spec_req_002_001
  tws_2 : ToWorkspace  VariableName=spec_req_002_002
  tws_3 : ToWorkspace  VariableName=spec_req_002_003
  result : Outport
  wires:
  sig_Req_Bus/1 -> BS_Req/1
  sig_Result_Bus/1 -> BS_Result/1
  AndN/1 -> result/1, result_tws/1
  BS_Req/1 -> cmp_1/1, Scope1/1  "<testSig_AccPed_stPTSLEna>"
  BS_Result/1 -> cmp_1/2, Scope1/2  "<AccPed_stPTSLEna>"
  cmp_1/1 -> Bitwise_And1/1
  Bitwise_And1/1 -> tws_1/1, AndN/1, Scope/1
  BS_Req/2 -> cmp_2/1, Scope2/1  "<testSig_AccPed_trqDes>"
  BS_Result/2 -> cmp_2/2, Scope2/2  "<AccPed_trqDes>"
  cmp_2/1 -> Bitwise_And2/1
  Bitwise_And2/1 -> tws_2/1, AndN/2, Scope/2
  BS_Req/3 -> cmp_3/1, Scope3/1  "<testSig_Epm_dnEng>"
  BS_Result/3 -> cmp_3/2, Scope3/2  "<Epm_dnEng>"
  cmp_3/1 -> Bitwise_And3/1
  Bitwise_And3/1 -> tws_3/1, AndN/3, Scope/3

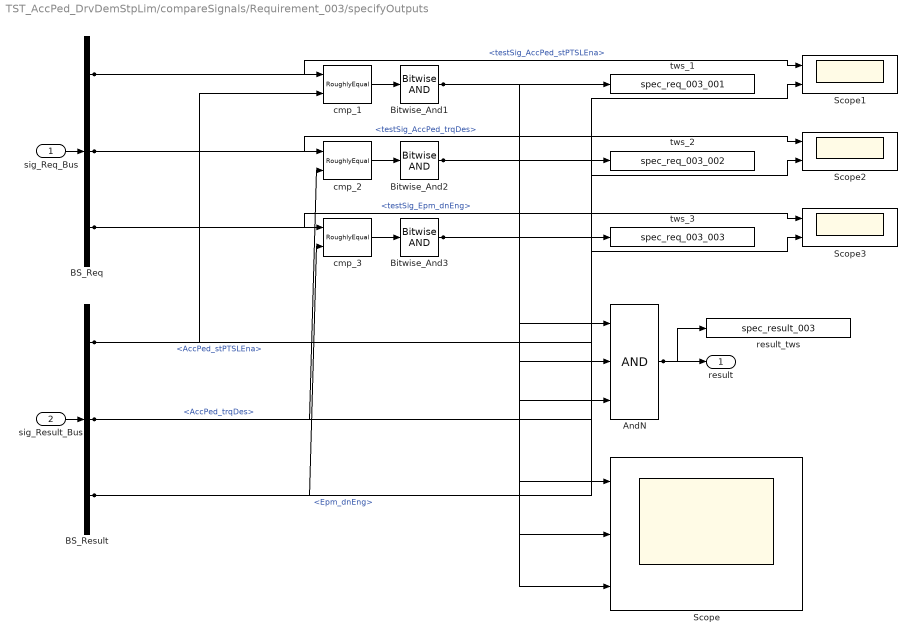
== system TST_AccPed_DrvDemStpLim/compareSignals/Requirement_003/specifyOutputs ==
  sig_Req_Bus : Inport
  sig_Result_Bus : Inport  Port=2
  AndN : Logic  Inputs=3
  BS_Req : BusSelector  OutputSignals=testSig_AccPed_stPTSLEna,testSig_AccPed_trqDes,testSig_Epm_dnEng
  BS_Result : BusSelector  OutputSignals=AccPed_stPTSLEna,AccPed_trqDes,Epm_dnEng
  Bitwise_And1 : simulink/Logic and Bit Operations/Bitwise Operator  logicop=AND  UseBitMask=off  BitMask=bin2dec('11011001')  BitMaskRealWorld=Stored Integer
  Bitwise_And2 : simulink/Logic and Bit Operations/Bitwise Operator  logicop=AND  UseBitMask=off  BitMask=bin2dec('11011001')  BitMaskRealWorld=Stored Integer
  Bitwise_And3 : simulink/Logic and Bit Operations/Bitwise Operator  logicop=AND  UseBitMask=off  BitMask=bin2dec('11011001')  BitMaskRealWorld=Stored Integer
  Scope : Scope  NumInputPorts=3
  Scope1 : Scope  NumInputPorts=2
  Scope2 : Scope  NumInputPorts=2
  Scope3 : Scope  NumInputPorts=2
  cmp_1 : UnitTest_Lib/RoughlyEqual  slope=0.1
  cmp_2 : UnitTest_Lib/RoughlyEqual  slope=0.1
  cmp_3 : UnitTest_Lib/RoughlyEqual  slope=0.1
  result_tws : ToWorkspace  VariableName=spec_result_003
  tws_1 : ToWorkspace  VariableName=spec_req_003_001
  tws_2 : ToWorkspace  VariableName=spec_req_003_002
  tws_3 : ToWorkspace  VariableName=spec_req_003_003
  result : Outport
  wires:
  sig_Req_Bus/1 -> BS_Req/1
  sig_Result_Bus/1 -> BS_Result/1
  AndN/1 -> result/1, result_tws/1
  BS_Req/1 -> cmp_1/1, Scope1/1  "<testSig_AccPed_stPTSLEna>"
  BS_Result/1 -> cmp_1/2, Scope1/2  "<AccPed_stPTSLEna>"
  cmp_1/1 -> Bitwise_And1/1
  Bitwise_And1/1 -> tws_1/1, AndN/1, Scope/1
  BS_Req/2 -> cmp_2/1, Scope2/1  "<testSig_AccPed_trqDes>"
  BS_Result/2 -> cmp_2/2, Scope2/2  "<AccPed_trqDes>"
  cmp_2/1 -> Bitwise_And2/1
  Bitwise_And2/1 -> tws_2/1, AndN/2, Scope/2
  BS_Req/3 -> cmp_3/1, Scope3/1  "<testSig_Epm_dnEng>"
  BS_Result/3 -> cmp_3/2, Scope3/2  "<Epm_dnEng>"
  cmp_3/1 -> Bitwise_And3/1
  Bitwise_And3/1 -> tws_3/1, AndN/3, Scope/3
